simulink model "msubsys2model7"  (Simulink 6.5)
settings: Solver=FixedStepDiscrete  StartTime=0.0  StopTime=10.0  RelTol=1e-3
settings Model: Creator=mani  LastModifiedBy=mani  ExtModeAutoUpdateStatusClock=off
settings DataIOCC: SaveFormat=Structure  OutputSaveName=yout1,yout2
settings OptimizationCC: OptimizeModelRefInitCode=on  LifeSpan=1
settings DebuggingCC: MultiTaskDSMMsg=warning  MultiTaskCondExecSysMsg=none
settings HardwareCC: TargetBitPerLong=64  TargetEndianess=LittleEndian  TargetWordSize=64  TargetHWDeviceType=MATLAB Host
settings RTWCC: SystemTargetFile=ert.tlc  TemplateMakefile=ert_default_tmf  Description=Real-Time Workshop Embedded Coder (no auto configuration)  RetainRTWFile=on  ProcessScript=ert_make_rtw_hook
settings CodeAppCC: IgnoreCustomStorageClasses=off
settings ERTTargetCC: TargetFcnLib=ansi_tfl_tmw.mat  GenFloatMathFcnCalls=ANSI_C  GenerateSampleERTMain=on  IncludeERTFirstTime=on  InlinedParameterPlacement=NonHierarchical  RTWCAPISignals=on  RTWCAPIParams=on  ERTCustomFileTemplate=example_file_process.tlc  InitialValueSource=Model

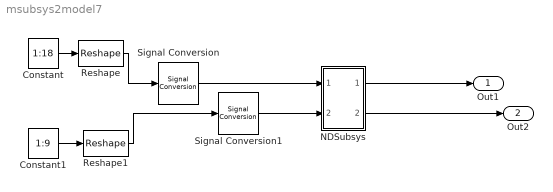
== system msubsys2model7 ==
  Constant : Constant  Value=1:18  SampleTime=1
  Constant1 : Constant  Value=1:9  SampleTime=1
  NDSubsys : Subsystem  TreatAsAtomicUnit=on
  Reshape : Reshape  OutputDimensionality=Customize (N-D)  OutputDimensions=[3 3 2]
  Reshape1 : Reshape  OutputDimensionality=Customize (N-D)  OutputDimensions=[3 1 1 3]
  Signal Conversion : SignalConversion  ConversionOutput=Contiguous copy  OverrideOpt=on
  Signal Conversion1 : SignalConversion  ConversionOutput=Contiguous copy  OverrideOpt=on
  Out1 : Outport
  Out2 : Outport  Port=2
  wires:
  Reshape1/1 -> Signal Conversion1/1
  NDSubsys/1(Out3) -> Out1/1
  NDSubsys/2(Out4) -> Out2/1
  Constant/1 -> Reshape/1
  Reshape/1 -> Signal Conversion/1
  Constant1/1 -> Reshape1/1
  Signal Conversion/1 -> NDSubsys/1(In1)
  Signal Conversion1/1 -> NDSubsys/2(In2)

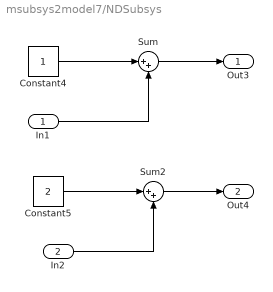
== system msubsys2model7/NDSubsys ==
  In1 : Inport  PortDimensions=[3 3 2]  Interpolate=off
  In2 : Inport  Port=2  PortDimensions=[3 1 1 3]  Interpolate=off
  Constant4 : Constant  SampleTime=1
  Constant5 : Constant  Value=2  SampleTime=1
  Sum : Sum  Inputs=|++
  Sum2 : Sum  Inputs=|++
  Out3 : Outport
  Out4 : Outport  Port=2
  wires:
  Constant4/1 -> Sum/1
  In1/1 -> Sum/2
  Sum/1 -> Out3/1
  Constant5/1 -> Sum2/1
  In2/1 -> Sum2/2
  Sum2/1 -> Out4/1
